simulink model "test_Arm"  (R2018a)
settings: Solver=VariableStepAuto  StartTime=0.0  StopTime=inf  RelTol=1e-3
libraries: simulink x6, sldrtlib x1
settings Model: Creator=tomato  LastModifiedBy=tomatoPC
settings CodeAppCC: StateflowObjectComments=on

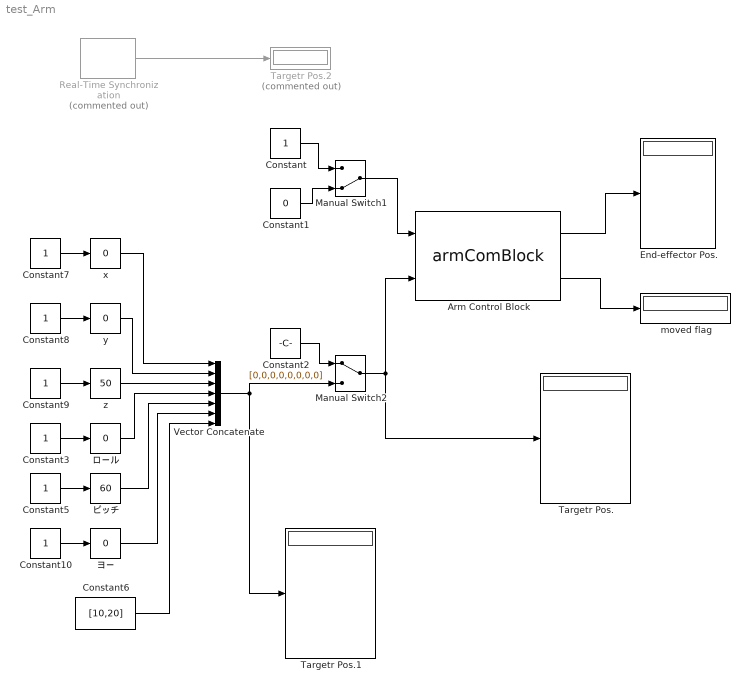
== system test_Arm ==
  Arm Control Block : M-S-Function  FunctionName=armComBlock  Parameters=comport, baud, tempPos  mask{comport='COM7', baud=115200, tempPos=[120,0,250,0,0,0,10,20]}
      mask prompts: comport "Port Number"; baud "Baudrate"; tempPos "Temporary Position"
      mask help: Canon Arm Control Block ver.0.8
      mask Display:
      | disp('Arm Control Block');
      | port_label('input',1,'Calib.');
      | port_label('input',2,'Target');
      | port_label('output',1,'Pos.');
      | port_label('output',2,'Moved');
  Constant{,3,5,7..10} (7 alike) : Constant
  Constant1 : Constant  Value=0
  Constant2 : Constant  Value=[0,0,0,0,0,0,0,0]
  Constant6 : Constant  Value=[10,20]
  End-effector Pos. : Display
  Manual Switch1 : ManualSwitch  CurrentSetting=0
  Manual Switch2 : ManualSwitch
  Real-Time Synchronization : sldrtlib/Real-Time Synchronization  Commented=on  SampleTime=0.1  MaxMissedTicks=inf  ShowMissedTicks=on  YieldWhenWaiting=off
  Targetr Pos. : Display
  Targetr Pos.1 : Display
  Targetr Pos.2 : Display  Commented=on
  Vector Concatenate : Concatenate  NumInputs=7
  moved flag : Display
  x : simulink/Math Operations/Slider Gain  gain=0  low=-500  high=500
  y : simulink/Math Operations/Slider Gain  gain=0  low=-100  high=100
  z : simulink/Math Operations/Slider Gain  gain=50  low=-100  high=100
  ピッチ : simulink/Math Operations/Slider Gain  gain=60  low=-100  high=100
  ヨー : simulink/Math Operations/Slider Gain  gain=0  low=-60  high=125
  ロール : simulink/Math Operations/Slider Gain  gain=0  low=-200  high=100
  wires:
  Arm Control Block/1 -> End-effector Pos./1
  Arm Control Block/2 -> moved flag/1
  Constant/1 -> Manual Switch1/1
  Constant1/1 -> Manual Switch1/2
  Manual Switch1/1 -> Arm Control Block/1
  Constant2/1 -> Manual Switch2/1
  Manual Switch2/1 -> Arm Control Block/2, Targetr Pos./1
  Constant7/1 -> x/1
  Constant8/1 -> y/1
  Constant9/1 -> z/1
  x/1 -> Vector Concatenate/1
  y/1 -> Vector Concatenate/2
  z/1 -> Vector Concatenate/3
  Vector Concatenate/1 -> Manual Switch2/2, Targetr Pos.1/1
  Real-Time Synchronization/1 -> Targetr Pos.2/1
  Constant10/1 -> ヨー/1
  ロール/1 -> Vector Concatenate/4
  Constant3/1 -> ロール/1
  ヨー/1 -> Vector Concatenate/6
  ピッチ/1 -> Vector Concatenate/5
  Constant5/1 -> ピッチ/1
  Constant6/1 -> Vector Concatenate/7
